simulink model "path_planning_test"  (R2020a)
settings: Solver=FixedStepAuto  StartTime=0.0  StopTime=inf  RelTol=1e-3
PreLoadFcn:
  | % ROS setup
  | rosshutdown;
  | ipAddr = '';
  | rosinit(ipAddr)
  | 
  | % Sample times
  | sampleTime = 0.2;
  | 
  | % Control parameters
  | ctrlParam1 = 2;
  | ctrlParam2 = 3.5;
undefined symbols (not defined in the file or in its folder): GpsCanLatitudeDegrees, GpsCanLongitudeDegrees, GpsCanTrueHeadingDegrees, par, WindSensor1AngleDegrees, WindSensor1SpeedKnots, WindSensor2AngleDegrees, WindSensor2SpeedKnots, WindSensor3AngleDegrees, WindSensor3SpeedKnots
libraries: robotlib x3, simulink_extras x3, UBCSailbotBlocks x2
settings Model: SimulationMode=external  Creator=scastro  LastModifiedBy=bruce
settings DataIOCC: ReturnWorkspaceOutputs=off
settings OptimizationCC: PassReuseOutputArgsAs=Individual arguments  MaxStackSize=64  EfficientTunableParamExpr=on
settings DebuggingCC: ParameterTunabilityLossMsg=error  ArithmeticOperatorsInVariantConditions=warning
settings HardwareCC: ProdBitPerLong=64  ProdHWDeviceType=Intel->x86-64 (Linux 64)
settings SFSimCC: SimUseLocalCustomCode=off  MATLABDynamicMemAlloc=off  CustomCodeUndefinedFunction=UseInterfaceOnly
settings RTWCC: SystemTargetFile=ert.tlc  HardwareBoard=Robot Operating System (ROS)  TemplateMakefile=ert_default_tmf  GenerateReport=on  RTWUseLocalCustomCode=off  Toolchain=Catkin  IncludeHyperlinkInReport=on  LaunchReport=on  PortableWordSizes=on  TargetLang=C++  GenerateTraceInfo=on  GenerateTraceReport=on  GenerateTraceReportSl=on  GenerateTraceReportSf=on  GenerateTraceReportEml=on
settings CodeAppCC: ForceParamTrailComments=on  IgnoreCustomStorageClasses=off  OperatorAnnotations=on  SimulinkDataObjDesc=on  SFDataObjDesc=on  InsertBlockDesc=on
settings ERTTargetCC: SupportContinuousTime=on  SupportVariableSizeSignals=on  ExtMode=on  ExtModeMexArgs='bruce-WS60-6QI' 0 17725

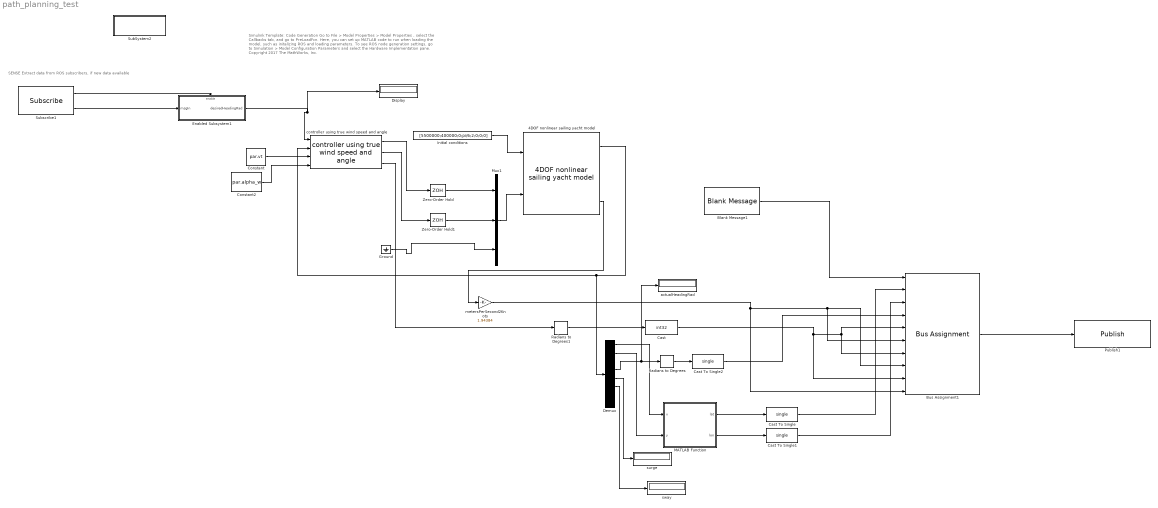
== system path_planning_test ==
  note: SENSE
      | Extract data from ROS subscribers, if new data available
  note: Simulink Template: Code Generation
      |
      | Go to File > Model Properties > Model Properties , select the Callbacks tab, and go to PreLoadFcn. Here, you can set up MATLAB code to run when loading the model, such as initalizing ROS and loading parameters.
      |
      | To see ROS node generation settings, go to Simulation > Model Configuration Parameters and select the Hardware Implementation pane.
      |
      | Copyright 2017 The MathWorks, Inc.
  4DOF nonlinear sailing yacht model : UBCSailbotBlocks/4DOF nonlinear sailing yacht model  SystemSampleTime=-1  Latency=0  AutoFrameSizeCalculation=off
  Blank Message1 : robotlib/Blank Message  messageClass=Message  entityType=sailbot_msg/Sensors  messageType=sailbot_msg/Sensors  SampleTime=inf
  Bus Assignment1 : BusAssignment  AssignedSignals=GpsCanLatitudeDegrees,GpsCanLongitudeDegrees,GpsCanTrueHeadingDegrees,WindSensor3AngleDegrees,WindSensor3SpeedKnots,WindSensor2AngleDegrees,WindSensor2SpeedKnots,WindSensor1AngleDegrees,WindSensor1SpeedKnots
  Cast : DataTypeConversion  OutDataTypeStr=int32
  Cast To Single : DataTypeConversion  OutDataTypeStr=single
  Cast To Single1 : DataTypeConversion  OutDataTypeStr=single
  Cast To Single2 : DataTypeConversion  OutDataTypeStr=single
  Constant : Constant  Value=par.vt
  Constant2 : Constant  Value=par.alpha_w  VectorParams1D=off
  Demux : Demux  Outputs=8
  Display : Display
  Enabled Subsystem1 : Subsystem  TreatAsAtomicUnit=on
  Ground : Ground
  Initial conditions : Constant  Value=[5500000;400000;0;pi/6;2;0;0;0]
  MATLAB Function : MATLAB Function  TreatAsAtomicUnit=on
  Mux1 : Mux  Inputs=3
  Publish1 : robotlib/Publish  topicSource=Specify your own  topic=/sensors  messageType=sailbot_msg/Sensors  messageQueueLength=1
  Radians to Degrees : simulink_extras/Transformations/Radians to Degrees
  Radians to Degrees1 : simulink_extras/Transformations/Radians to Degrees
  SubSystem2 : Subsystem  InitFcn=|
      | global par
      | par.m = 25900;                         % (kg),mass of the vehicle
      | par.Ixx = 133690;          
      | par.Izz = 24760;      
      | par.Ixz = 2180;                        % moment of inertia
      | par.a11 = 970;   
      | par.a22 = 17430; 
      | par.a44 = 106500;
      | par.a66 = 101650;
      | par.a24 = -13160;
      | par.a26 = -6190; 
      | par.a46 = 4730;                        % (kg),added mass coef.
      | 
      | par.vt = 5;                           % the norm of wind velocity
      | par.alpha_w = pi/4;                      % the direction of wind (coming from the north, ie going south)
      | 
      | par.rho_a = 1.2;                       % (kg/m^3), air density
      | par.As = 170;                          % (m^2), sail area
      | par.h0 = 0.0005;                       % (m), roughness height
      | par.h1 = 11.58;                        % (m), reference height
      | par.z_s = -11.58;                      % (m), (x,y,z) is the CoE
      | par.xs = 0;
      | par.ys = 0;
      | par.zs = -11.58;                       % (m), (x,y,z) is the CoE
      | par.Xce = 0.6;                         % (m), distance along the mast to the CoE
      | par.Xm = 0.3;                          % (m), x-coordinate of the mast 
      | 
      | par.rho_w = 1025;                      % (kg/m^3), water density
      | par.Ar = 1.17;                         % (m^2), rudder area
      | par.d_r = 1.9;                         % rudder draft
      | par.zeta_r = 0.8;                      % rudder efficiency
      | par.x_r = -8.2;
      | par.z_r = -0.78;                       % (m), (x,y,z) is the CoE
      | par.xr = -8.2;
      | par.yr = 0;
      | par.zr = -0.78;                        % (m), (x,y,z) is the CoE
      | 
      | par.Ak = 8.7;                          % (m^2), keel area
      | par.d_k = 2.49;                        % keel draft
      | par.zeta_k = 0.7;                      % keel efficiency
      | par.x_k = 0;
      | par.z_k = -0.58;                       % (m), (x,y,z) is the CoE
      | par.xk = 0;
      | par.yk = 0;
      | par.zk = -0.58;                        % (m), (x,y,z) is the CoE
      | 
      | par.x_h = 0;
      | par.z_h = -1.18;                       % (m), (x,y,z) is the CoE
      | par.xh = 0;
      | par.yh = 0;
      | par.zh = -1.18;                        % (m), (x,y,z) is the CoE
      | 
      | par.w_c = 60000;                       % (N), crew weight 20000
      | par.x_c = -8;                          % (m), crew position
      | par.y_bm = 3.6;                        % (m), yacht beam
      | 
      | par.a = -5.89;
      | par.b = 8160;
      | par.c = 120000;
      | par.d = 50000;
      mask Display: disp('Parameter Initialization')
  Subscribe1 : robotlib/Subscribe  topicSource=Specify your own  topic=/heading_degrees  messageType=sailbot_msg/heading  sampleTime=-1  messageQueueLength=1
  Zero-Order Hold : ZeroOrderHold  SampleTime=0.1
  Zero-Order Hold1 : ZeroOrderHold  SampleTime=0.1
  actualHeadingRad : Display
  controller using true wind speed and angle : UBCSailbotBlocks/controller using true wind speed and angle  SystemSampleTime=-1  Latency=0  AutoFrameSizeCalculation=off
  metersPerSecond2Knots : Gain  Gain=1.94384  OutDataTypeStr=single
  surge : Display
  sway : Display
  wires:
  Subscribe1/2 -> Enabled Subsystem1/1(msgIn)
  controller using true wind speed and angle/1 -> Zero-Order Hold/1
  Subscribe1/1 -> Enabled Subsystem1/Enable
  Bus Assignment1/1 -> Publish1/1
  4DOF nonlinear sailing yacht model/1 -> Demux/1, controller using true wind speed and angle/2
  Initial conditions/1 -> 4DOF nonlinear sailing yacht model/1
  Blank Message1/1 -> Bus Assignment1/1
  Mux1/1 -> 4DOF nonlinear sailing yacht model/2
  Constant2/1 -> controller using true wind speed and angle/4
  controller using true wind speed and angle/2 -> Zero-Order Hold1/1
  Demux/1 -> MATLAB Function/1(x)
  Demux/2 -> MATLAB Function/2(y)
  Zero-Order Hold/1 -> Mux1/1
  Zero-Order Hold1/1 -> Mux1/2
  Ground/1 -> Mux1/3
  Constant/1 -> controller using true wind speed and angle/3
  controller using true wind speed and angle/3 -> Radians to Degrees1/1
  Demux/4 -> Radians to Degrees/1, actualHeadingRad/1
  Enabled Subsystem1/1(desiredHeadingRad) -> Display/1, controller using true wind speed and angle/1
  Radians to Degrees1/1 -> Cast/1
  4DOF nonlinear sailing yacht model/3 -> metersPerSecond2Knots/1
  MATLAB Function/1(lat) -> Cast To Single/1
  MATLAB Function/2(lon) -> Cast To Single1/1
  Radians to Degrees/1 -> Cast To Single2/1
  Cast/1 -> Bus Assignment1/9, Bus Assignment1/5, Bus Assignment1/7
  metersPerSecond2Knots/1 -> Bus Assignment1/10, Bus Assignment1/6, Bus Assignment1/8
  Cast To Single/1 -> Bus Assignment1/2
  Cast To Single1/1 -> Bus Assignment1/3
  Cast To Single2/1 -> Bus Assignment1/4
  Demux/5 -> surge/1
  Demux/6 -> sway/1

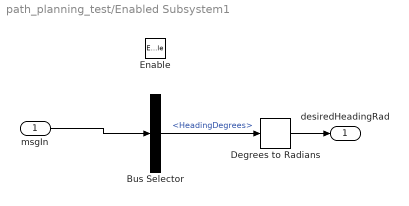
== system path_planning_test/Enabled Subsystem1 ==
  msgIn : Inport
  Enable : EnablePort
  Bus Selector : BusSelector  OutputSignals=HeadingDegrees
  Degrees to Radians : simulink_extras/Transformations/Degrees to Radians
  desiredHeadingRad : Outport  VectorParamsAs1DForOutWhenUnconnected=off
  wires:
  msgIn/1 -> Bus Selector/1
  Bus Selector/1 -> Degrees to Radians/1  "<HeadingDegrees>"
  Degrees to Radians/1 -> desiredHeadingRad/1

== system path_planning_test/SubSystem2 ==

== matlab function path_planning_test/MATLAB Function ==
  data: x input; lat output; y input; lon output
function [lat, lon] = metersToLatLonWrapper(x, y)
coder.extrinsic('metersToLatLon'); 
lat = NaN;
lon = NaN;
[lat,lon] = metersToLatLon(x,y);
